simulink model "quadcopter"  (R2019b)
settings: Solver=VariableStepAuto  StartTime=0.0  StopTime=10.0  RelTol=1e-3
values from neighbouring files (symbols this model uses):
  An = 0.25    [constants_drone.m]
  b = 3.0 *10^-5    (= 3e-05)    [constants_drone.m]    (also in drone.m)
  d = 1.1*10^-6    (= 1.1e-06)    [constants_drone.m]    (also in drone.m)
  Ixx = 6.12*10^-2    (= 0.0612)    [constants_drone.m]
  Iyy = Ixx    (= 0.0612)    [constants_drone.m]
  Izz = 8.11*10^-2    (= 0.0811)    [constants_drone.m]
  Jr = (1/2)*(m*0.01^2)    (= 2.5e-05)    [constants_drone.m]    (also in drone.m = 0.001)
  l = 0.225    [constants_drone.m]    (also in drone.m = 0.25)
  m = 0.5    [constants_drone.m]    (also in drone.m; drone_test.m = 0.25)
  omega1 = 220    [constants_drone.m]
  omega2 = 219    [constants_drone.m]
  omega3 = 220    [constants_drone.m]
  omega4 = 220    [constants_drone.m]
settings Model: Creator=Emil  LastModifiedBy=Emil
settings DebuggingCC: UnderSpecifiedDimensionMsg=warning

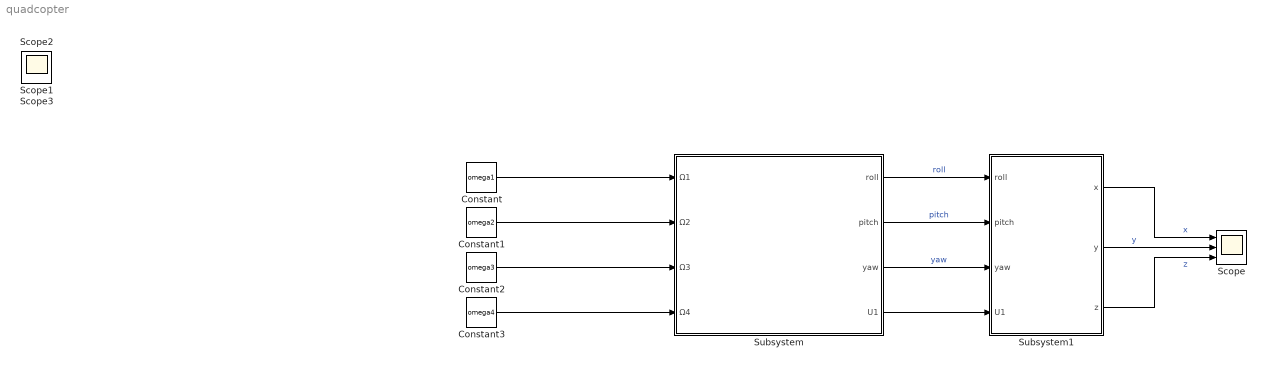
== system quadcopter ==
  Constant : Constant  Value=omega1
  Constant1 : Constant  Value=omega2
  Constant2 : Constant  Value=omega3
  Constant3 : Constant  Value=omega4
  Scope : Scope  NumInputPorts=3
  Subsystem : Subsystem
  Subsystem1 : Subsystem
  Scope1 : Scope
  Scope2 : Scope
  Scope3 : Scope
  wires:
  Subsystem/3(yaw) -> Subsystem1/3(yaw)  "yaw"
  Subsystem/2(pitch) -> Subsystem1/2(pitch)  "pitch"
  Subsystem/1(roll) -> Subsystem1/1(roll)  "roll"
  Subsystem/4(U1) -> Subsystem1/4(U1)
  Subsystem1/2(y) -> Scope/2  "y"
  Subsystem1/1(x) -> Scope/1  "x"
  Subsystem1/3(z) -> Scope/3  "z"
  Constant/1 -> Subsystem/1(Ω1)
  Constant1/1 -> Subsystem/2(Ω2)
  Constant2/1 -> Subsystem/3(Ω3)
  Constant3/1 -> Subsystem/4(Ω4)

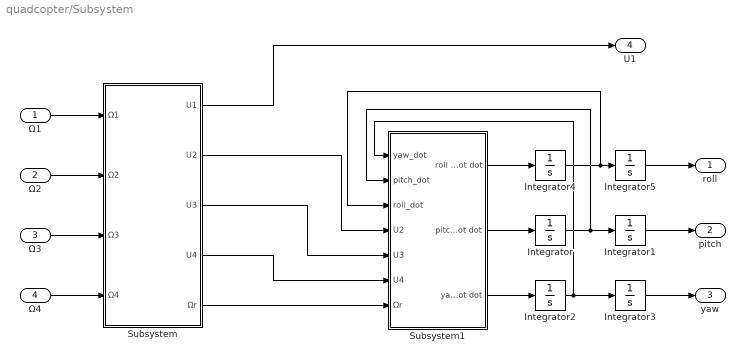
== system quadcopter/Subsystem ==
  Ω1 : Inport
  Ω2 : Inport  Port=2
  Ω3 : Inport  Port=3
  Ω4 : Inport  Port=4
  Integrator : Integrator
  Integrator1 : Integrator  WrapState=on
  Integrator2 : Integrator
  Integrator3 : Integrator  WrapState=on
  Integrator4 : Integrator
  Integrator5 : Integrator  WrapState=on
  Subsystem : Subsystem
  Subsystem1 : Subsystem
  roll : Outport
  pitch : Outport  Port=2
  yaw : Outport  Port=3
  U1 : Outport  Port=4
  wires:
  Ω1/1 -> Subsystem/1(Ω1)
  Ω2/1 -> Subsystem/2(Ω2)
  Ω3/1 -> Subsystem/3(Ω3)
  Ω4/1 -> Subsystem/4(Ω4)
  Subsystem/2(U2) -> Subsystem1/4(U2)
  Subsystem/3(U3) -> Subsystem1/5(U3)
  Subsystem/4(U4) -> Subsystem1/6(U4)
  Subsystem/5(Ωr) -> Subsystem1/7(Ωr)
  Subsystem1/2(pitch dot dot) -> Integrator/1
  Integrator/1 -> Subsystem1/2(pitch_dot), Integrator1/1
  Subsystem1/3(yaw dot dot) -> Integrator2/1
  Integrator2/1 -> Subsystem1/1(yaw_dot), Integrator3/1
  Subsystem1/1(roll dot dot) -> Integrator4/1
  Integrator4/1 -> Subsystem1/3(roll_dot), Integrator5/1
  Integrator5/1 -> roll/1
  Integrator1/1 -> pitch/1
  Integrator3/1 -> yaw/1
  Subsystem/1(U1) -> U1/1

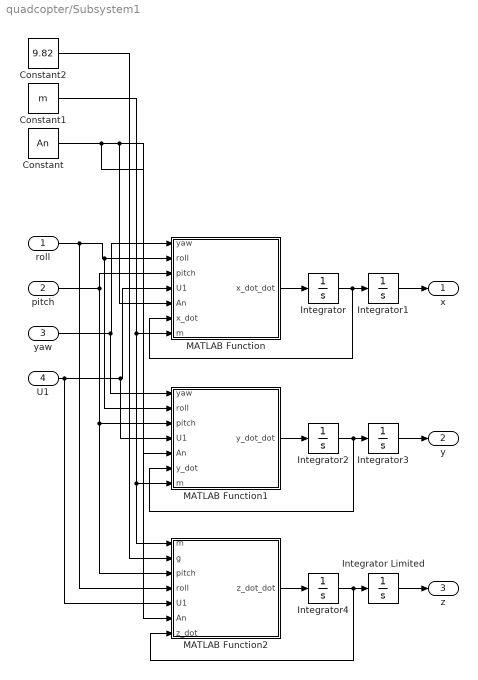
== system quadcopter/Subsystem1 ==
  roll : Inport
  pitch : Inport  Port=2
  yaw : Inport  Port=3
  U1 : Inport  Port=4
  Constant : Constant  Value=An
  Constant1 : Constant  Value=m
  Constant2 : Constant  Value=9.82
  Integrator{,1..4} (5 alike) : Integrator
  Integrator Limited : Integrator  UpperSaturationLimit=0
  MATLAB Function : MATLAB Function  TreatAsAtomicUnit=on
  MATLAB Function1 : MATLAB Function  TreatAsAtomicUnit=on
  MATLAB Function2 : MATLAB Function  TreatAsAtomicUnit=on
  x : Outport
  y : Outport  Port=2
  z : Outport  Port=3
  wires:
  roll/1 -> MATLAB Function1/2(roll), MATLAB Function/2(roll), MATLAB Function2/4(roll)
  pitch/1 -> MATLAB Function2/3(pitch), MATLAB Function1/3(pitch), MATLAB Function/3(pitch)
  yaw/1 -> MATLAB Function1/1(yaw), MATLAB Function/1(yaw)
  U1/1 -> MATLAB Function2/5(U1), MATLAB Function1/4(U1), MATLAB Function/4(U1)
  Constant/1 -> MATLAB Function2/6(An), MATLAB Function1/5(An), MATLAB Function/5(An)
  MATLAB Function/1(x_dot_dot) -> Integrator/1
  Integrator1/1 -> x/1
  Integrator/1 -> MATLAB Function/6(x_dot), Integrator1/1
  MATLAB Function1/1(y_dot_dot) -> Integrator2/1
  Integrator2/1 -> MATLAB Function1/6(y_dot), Integrator3/1
  Integrator3/1 -> y/1
  Constant1/1 -> MATLAB Function2/1(m), MATLAB Function1/7(m), MATLAB Function/7(m)
  Constant2/1 -> MATLAB Function2/2(g)
  Integrator4/1 -> Integrator Limited/1, MATLAB Function2/7(z_dot)
  Integrator Limited/1 -> z/1
  MATLAB Function2/1(z_dot_dot) -> Integrator4/1

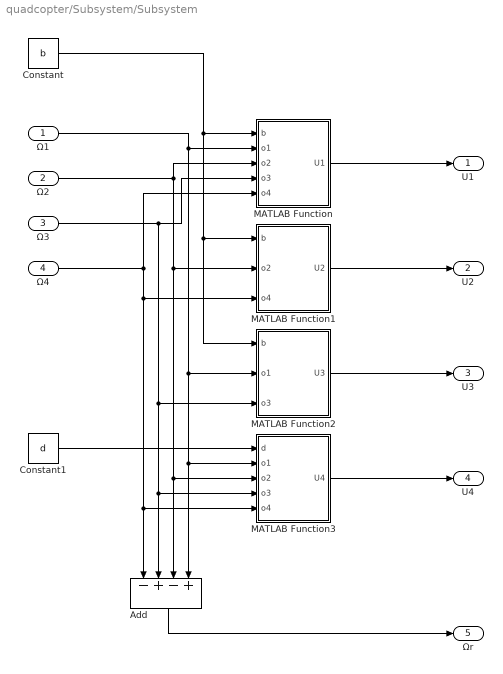
== system quadcopter/Subsystem/Subsystem ==
  Ω1 : Inport
  Ω2 : Inport  Port=2
  Ω3 : Inport  Port=3
  Ω4 : Inport  Port=4
  Add : Sum  Inputs=-+-+
  Constant : Constant  Value=b
  Constant1 : Constant  Value=d
  MATLAB Function : MATLAB Function  TreatAsAtomicUnit=on
  MATLAB Function1 : MATLAB Function  TreatAsAtomicUnit=on
  MATLAB Function2 : MATLAB Function  TreatAsAtomicUnit=on
  MATLAB Function3 : MATLAB Function  TreatAsAtomicUnit=on
  U1 : Outport
  U2 : Outport  Port=2
  U3 : Outport  Port=3
  U4 : Outport  Port=4
  Ωr : Outport  Port=5
  wires:
  Add/1 -> Ωr/1
  Ω4/1 -> MATLAB Function1/3(o4), MATLAB Function3/5(o4), Add/1, MATLAB Function/5(o4)
  Ω3/1 -> MATLAB Function2/3(o3), MATLAB Function3/4(o3), Add/2, MATLAB Function/4(o3)
  Ω2/1 -> MATLAB Function/3(o2), MATLAB Function1/2(o2), MATLAB Function3/3(o2), Add/3
  Ω1/1 -> MATLAB Function2/2(o1), MATLAB Function3/2(o1), Add/4, MATLAB Function/2(o1)
  MATLAB Function/1(U1) -> U1/1
  MATLAB Function1/1(U2) -> U2/1
  MATLAB Function2/1(U3) -> U3/1
  MATLAB Function3/1(U4) -> U4/1
  Constant/1 -> MATLAB Function2/1(b), MATLAB Function1/1(b), MATLAB Function/1(b)
  Constant1/1 -> MATLAB Function3/1(d)

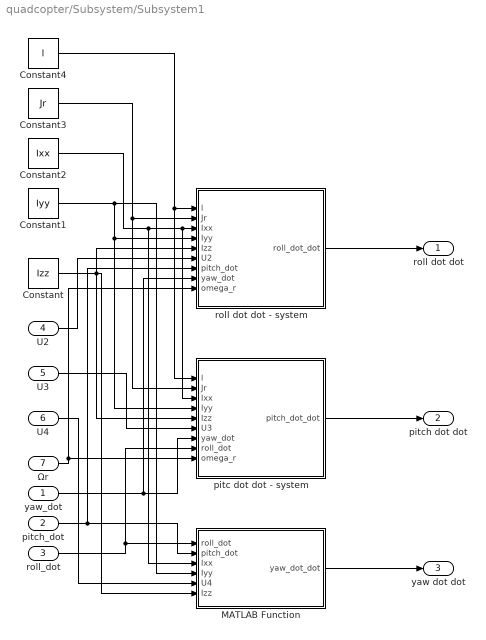
== system quadcopter/Subsystem/Subsystem1 ==
  yaw_dot : Inport
  pitch_dot : Inport  Port=2
  roll_dot : Inport  Port=3
  U2 : Inport  Port=4
  U3 : Inport  Port=5
  U4 : Inport  Port=6
  Ωr : Inport  Port=7
  Constant : Constant  Value=Izz
  Constant1 : Constant  Value=Iyy
  Constant2 : Constant  Value=Ixx
  Constant3 : Constant  Value=Jr
  Constant4 : Constant  Value=l
  MATLAB Function : MATLAB Function  TreatAsAtomicUnit=on
  pitc dot dot - system : MATLAB Function  TreatAsAtomicUnit=on
  "roll dot dot - system " : MATLAB Function  TreatAsAtomicUnit=on
  roll dot dot : Outport
  pitch dot dot : Outport  Port=2
  yaw dot dot : Outport  Port=3
  wires:
  U2/1 -> "roll dot dot - system "/6(U2)
  Constant3/1 -> pitc dot dot - system/2(Jr), "roll dot dot - system "/2(Jr)
  Constant2/1 -> MATLAB Function/3(Ixx), pitc dot dot - system/3(Ixx), "roll dot dot - system "/3(Ixx)
  Constant1/1 -> MATLAB Function/4(Iyy), pitc dot dot - system/4(Iyy), "roll dot dot - system "/4(Iyy)
  Constant/1 -> MATLAB Function/6(Izz), "roll dot dot - system "/5(Izz), pitc dot dot - system/5(Izz)
  "roll dot dot - system "/1(roll_dot_dot) -> roll dot dot/1
  pitc dot dot - system/1(pitch_dot_dot) -> pitch dot dot/1
  MATLAB Function/1(yaw_dot_dot) -> yaw dot dot/1
  Ωr/1 -> "roll dot dot - system "/9(omega_r), pitc dot dot - system/9(omega_r)
  U3/1 -> pitc dot dot - system/6(U3)
  Constant4/1 -> "roll dot dot - system "/1(l), pitc dot dot - system/1(l)
  U4/1 -> MATLAB Function/5(U4)
  pitch_dot/1 -> MATLAB Function/2(pitch_dot), "roll dot dot - system "/7(pitch_dot)
  yaw_dot/1 -> "roll dot dot - system "/8(yaw_dot), pitc dot dot - system/7(yaw_dot)
  roll_dot/1 -> MATLAB Function/1(roll_dot), pitc dot dot - system/8(roll_dot)

== matlab function quadcopter/Subsystem/Subsystem/MATLAB Function1 ==
  data: b input; U2 output; o2 input; o4 input
function U2 = fcn(b, o2, o4)

U2 = b*(-o2^2+o4^2);

== matlab function quadcopter/Subsystem/Subsystem/MATLAB Function ==
  data: b input; U1 output; o1 input; o2 input; o3 input; o4 input
function U1 = fcn(b, o1, o2, o3, o4)

U1 = b*(o1^2+o2^2+o3^2+o4^2);

== matlab function quadcopter/Subsystem/Subsystem/MATLAB Function2 ==
  data: b input; U3 output; o1 input; o3 input
function U3 = fcn(b, o1, o3)

U3 = b*(o1^2-o3^2);

== matlab function quadcopter/Subsystem/Subsystem/MATLAB Function3 ==
  data: d input; U4 output; o1 input; o2 input; o3 input; o4 input
function U4 = fcn(d, o1, o2, o3, o4)

U4 = d*(o1^2-o2^2+o3^2-o4^2);

== matlab function quadcopter/Subsystem/Subsystem1/roll dot dot - system  ==
  data: l input; Jr input; Ixx input; Iyy input; Izz input; roll_dot_dot output; U2 input; pitch_dot input; yaw_dot input; omega_r input
function roll_dot_dot = fcn(l, Jr, Ixx, Iyy, Izz, U2,pitch_dot , yaw_dot, omega_r)

roll_dot_dot = pitch_dot*yaw_dot*((Iyy-Izz)/Ixx)+(1/Ixx)*U2;

== matlab function quadcopter/Subsystem/Subsystem1/pitc dot dot - system ==
  data: l input; Jr input; Ixx input; Iyy input; Izz input; pitch_dot_dot output; U3 input; yaw_dot input; roll_dot input; omega_r input
function pitch_dot_dot = fcn(l, Jr, Ixx, Iyy, Izz, U3, yaw_dot, roll_dot, omega_r)

pitch_dot_dot = roll_dot*yaw_dot*((Izz-Ixx)/Iyy)+(1/Iyy)*U3;

== matlab function quadcopter/Subsystem/Subsystem1/MATLAB Function ==
  data: roll_dot input; yaw_dot_dot output; pitch_dot input; Ixx input; Iyy input; U4 input; Izz input
function yaw_dot_dot = fcn(roll_dot, pitch_dot, Ixx, Iyy, U4, Izz)

yaw_dot_dot = pitch_dot*roll_dot*((Ixx-Iyy)/Izz)+(1/Izz)*U4;

== matlab function quadcopter/Subsystem1/MATLAB Function ==
  data: yaw input; roll input; pitch input; U1 input; An input; x_dot input; x_dot_dot output; m input
function x_dot_dot = fcn(yaw, roll, pitch, U1, An, x_dot, m)


x_dot_dot = (0.9*pitch)*(U1/m);

== matlab function quadcopter/Subsystem1/MATLAB Function1 ==
  data: yaw input; roll input; pitch input; U1 input; An input; y_dot input; y_dot_dot output; m input
function y_dot_dot = fcn(yaw, roll, pitch, U1, An, y_dot, m)

y_dot_dot = (-0.95*roll)*(U1/m);

== matlab function quadcopter/Subsystem1/MATLAB Function2 ==
  data: m input; z_dot_dot output; g input; pitch input; roll input; U1 input; An input; z_dot input
function z_dot_dot = fcn(m, g, pitch, roll, U1, An, z_dot)

z_dot_dot = -g+0.9*(U1/m);
